simulink model "Controle_nivel_tanque"  (R2016a)
settings: Solver=VariableStepAuto  StartTime=0.0  StopTime=inf  RelTol=1e-3
undefined symbols (not defined in the file or in its folder): A, p, q
libraries: simulink x1
settings Model: Creator=Vitor  LastModifiedBy=Vitor

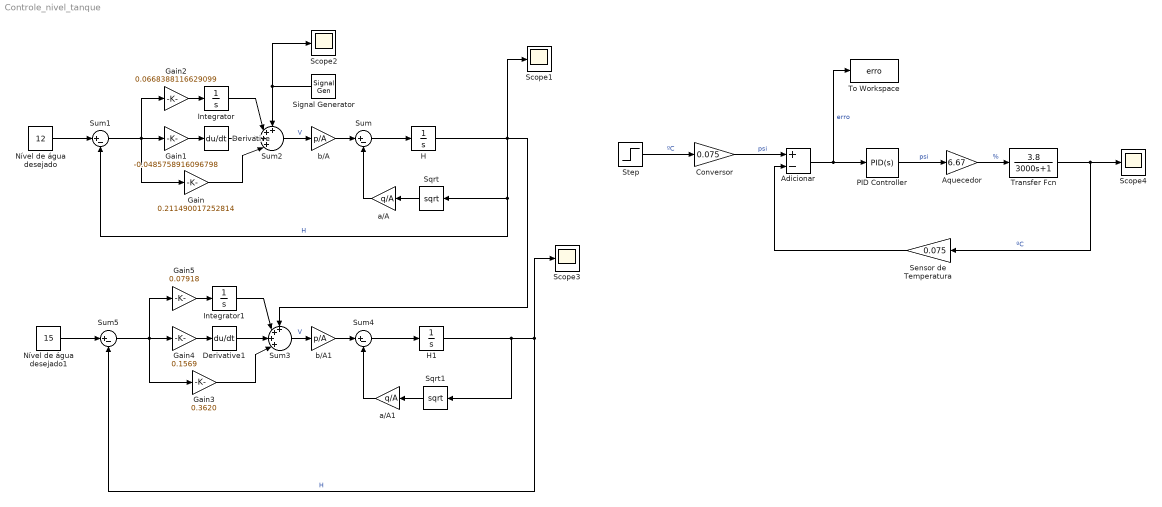
== system Controle_nivel_tanque ==
  "Adicionar " : Sum  Inputs=+-
  "Aquecedor " : Gain  Gain=6.67
  "Conversor " : Gain  Gain=0.075
  Derivative : Derivative
  Derivative1 : Derivative
  Gain : Gain  Gain=0.211490017252814
  Gain1 : Gain  Gain=-0.0485758916096798
  Gain2 : Gain  Gain=0.0668388116629099
  Gain3 : Gain  Gain=0.3620
  Gain4 : Gain  Gain=0.1569
  Gain5 : Gain  Gain=0.07918
  H : Integrator  InitialCondition=10
  H1 : Integrator  InitialCondition=10
  Integrator : Integrator
  Integrator1 : Integrator
  Nível de água desejado : Constant  Value=12
  Nível de água desejado1 : Constant  Value=15
  PID Controller : simulink/Continuous/PID Controller  Controller=PID  TimeDomain=Continuous-time  SampleTime=-1  IntegratorMethod=Forward Euler  FilterMethod=Forward Euler  Form=Parallel  UseFilter=on  ControllerParametersSource=internal  P=0.703637819929562  I=0.000468809887414056  D=-76.6604460028091  N=0.00126031388394287  InitialConditionSource=internal  InitialConditionForIntegrator=0  InitialConditionForFilter=0  ExternalReset=none  LimitOutput=off  UpperSaturationLimit=inf  LowerSaturationLimit=-inf  LinearizeAsGain=on  AntiWindupMode=none  Kb=1  TrackingMode=off  Kt=1  PParamMin=[]  PParamMax=[]  IParamMin=[]  IParamMax=[]  DParamMin=[]  DParamMax=[]  NParamMin=[]  NParamMax=[]  KbParamMin=[]  KbParamMax=[]  KtParamMin=[]  KtParamMax=[]  POutMin=[]  POutMax=[]  IOutMin=[]  IOutMax=[]  DOutMin=[]  DOutMax=[]  NOutMin=[]  NOutMax=[]  KbOutMin=[]  KbOutMax=[]  KtOutMin=[]  KtOutMax=[]  IntegratorOutMin=[]  IntegratorOutMax=[]  FilterOutMin=[]  FilterOutMax=[]  SumOutMin=[]  SumOutMax=[]  SumI1OutMin=[]  SumI1OutMax=[]  SumI2OutMin=[]  SumI2OutMax=[]  SumI3OutMin=[]  SumI3OutMax=[]  SumDOutMin=[]  SumDOutMax=[]  SaturationOutMin=[]  SaturationOutMax=[]  IntegratorContinuousStateAttributes=''  IntegratorStateMustResolveToSignalObject=off  IntegratorRTWStateStorageClass=Auto  FilterContinuousStateAttributes=''  FilterStateMustResolveToSignalObject=off  FilterRTWStateStorageClass=Auto  DifferentiatorICPrevScaledInput=0  DifferentiatorOutMin=[]  DifferentiatorOutMax=[]
  Scope{1..4} (4 alike) : Scope
  "Sensor de Temperatura " : Gain  Gain=0.075
  Signal Generator : SignalGenerator  Amplitude=0.1  Frequency=0.03  Units=rad/sec
  Sqrt : Sqrt  SaturateOnIntegerOverflow=on
  Sqrt1 : Sqrt  SaturateOnIntegerOverflow=on
  Step : Step  Before=10  After=10000  SampleTime=0
  Sum{,1,4..5} (4 alike) : Sum  Inputs=|+-  SaturateOnIntegerOverflow=on
  Sum2 : Sum  Inputs=++++|
  Sum3 : Sum  Inputs=++++|
  To Workspace : ToWorkspace  VariableName=erro  SaveFormat=Timeseries  SampleTime=-1
  Transfer Fcn : TransferFcn  Numerator=[3.8]  Denominator=[3000 1]
  a/A : Gain  Gain=q/A  SaturateOnIntegerOverflow=on  OutDataTypeStr=Inherit: Same as input  ParamDataTypeStr=Inherit: Same as input
  a/A1 : Gain  Gain=q/A  SaturateOnIntegerOverflow=on  OutDataTypeStr=Inherit: Same as input  ParamDataTypeStr=Inherit: Same as input
  b/A : Gain  Gain=p/A  SaturateOnIntegerOverflow=on  OutDataTypeStr=Inherit: Same as input  ParamDataTypeStr=Inherit: Same as input
  b/A1 : Gain  Gain=p/A  SaturateOnIntegerOverflow=on  OutDataTypeStr=Inherit: Same as input  ParamDataTypeStr=Inherit: Same as input
  wires:
  Nível de água desejado/1 -> Sum1/1
  Nível de água desejado1/1 -> Sum5/1
  Derivative/1 -> Sum2/3
  Integrator/1 -> Sum2/2
  Gain1/1 -> Derivative/1
  Gain2/1 -> Integrator/1
  Sum1/1 -> Gain2/1, Gain1/1, Gain/1
  Signal Generator/1 -> Sum2/1, Scope2/1
  b/A/1 -> Sum/1
  Sum/1 -> H/1
  H/1 -> Sum1/2, Sqrt/1, Sum3/1, Scope1/1  "H"
  Sqrt/1 -> a/A/1
  a/A/1 -> Sum/2
  Sum2/1 -> b/A/1  "V"
  Gain3/1 -> Sum3/4
  Derivative1/1 -> Sum3/3
  Integrator1/1 -> Sum3/2
  Gain4/1 -> Derivative1/1
  Gain5/1 -> Integrator1/1
  Sum5/1 -> Gain5/1, Gain4/1, Gain3/1
  b/A1/1 -> Sum4/1
  Sum4/1 -> H1/1
  H1/1 -> Sqrt1/1, Sum5/2, Scope3/1  "H"
  Sqrt1/1 -> a/A1/1
  a/A1/1 -> Sum4/2
  Sum3/1 -> b/A1/1  "V"
  Gain/1 -> Sum2/4
  "Sensor de Temperatura "/1 -> "Adicionar "/2
  "Conversor "/1 -> "Adicionar "/1  "psi"
  "Adicionar "/1 -> To Workspace/1, PID Controller/1  "erro"
  PID Controller/1 -> "Aquecedor "/1  "psi"
  "Aquecedor "/1 -> Transfer Fcn/1  "%"
  Transfer Fcn/1 -> "Sensor de Temperatura "/1, Scope4/1  "ºC"
  Step/1 -> "Conversor "/1  "ºC"
